simulink model "carKinematicSimulator"  (R2025b)
settings: Solver=VariableStepAuto  StartTime=0.0  StopTime=10.0  RelTol=1e-3
settings Model: Creator=sprinkle  LastModifiedBy=sprinkle

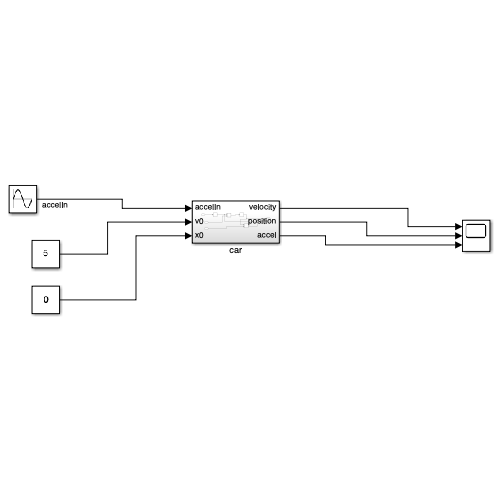
[thumbnail: Simulink's stored preview of the top-level diagram]
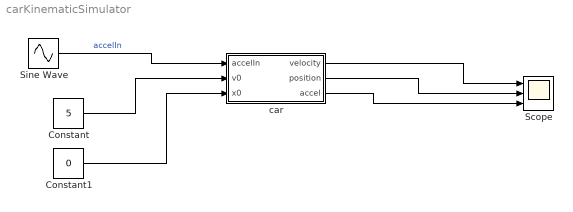
== system carKinematicSimulator ==
  Constant : Constant  Value=5
  Constant1 : Constant  Value=0
  Scope : Scope  NumInputPorts=3
      settings: ActiveDisplayYMinimum=-9.6431780692017686  ActiveDisplayYMaximum=51.788602622815922
  Sine Wave : Sin  Amplitude=10  SampleTime=0
  car : Subsystem
  wires:
  Sine Wave/1 -> car/1(accelIn)  "accelIn"
  Constant/1 -> car/2(v0)
  Constant1/1 -> car/3(x0)
  car/1(velocity) -> Scope/1
  car/2(position) -> Scope/2
  car/3(accel) -> Scope/3

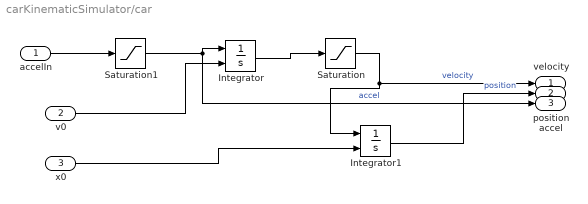
== system carKinematicSimulator/car ==
  accelIn : Inport
  v0 : Inport  Port=2
  x0 : Inport  Port=3
  Integrator : Integrator  InitialConditionSource=external
  Integrator1 : Integrator  InitialConditionSource=external
  Saturation : Saturate  UpperLimit=30  LowerLimit=0
  Saturation1 : Saturate  UpperLimit=1.5  LowerLimit=-3.5
  velocity : Outport
  position : Outport  Port=2
  accel : Outport  Port=3
  wires:
  x0/1 -> Integrator1/2
  Integrator1/1 -> position/1  "position"
  Saturation/1 -> velocity/1, Integrator1/1  "velocity"
  v0/1 -> Integrator/2
  accelIn/1 -> Saturation1/1
  Integrator/1 -> Saturation/1
  Saturation1/1 -> accel/1, Integrator/1  "accel"
